simulink model "fullSys"  (R2013a)
settings: Solver=ode45  StartTime=0.0  StopTime=10.0  RelTol=1e-3
values from neighbouring files (symbols this model uses):
  g = 9.81    [init.m]
  I = diag([4.856e-3,4.856e-3,8.801e-3])    [init.m]
  m = 0.468    [init.m]
libraries: simulink x1
settings Model: Creator=vegardvo  LastModifiedBy=vegardvo

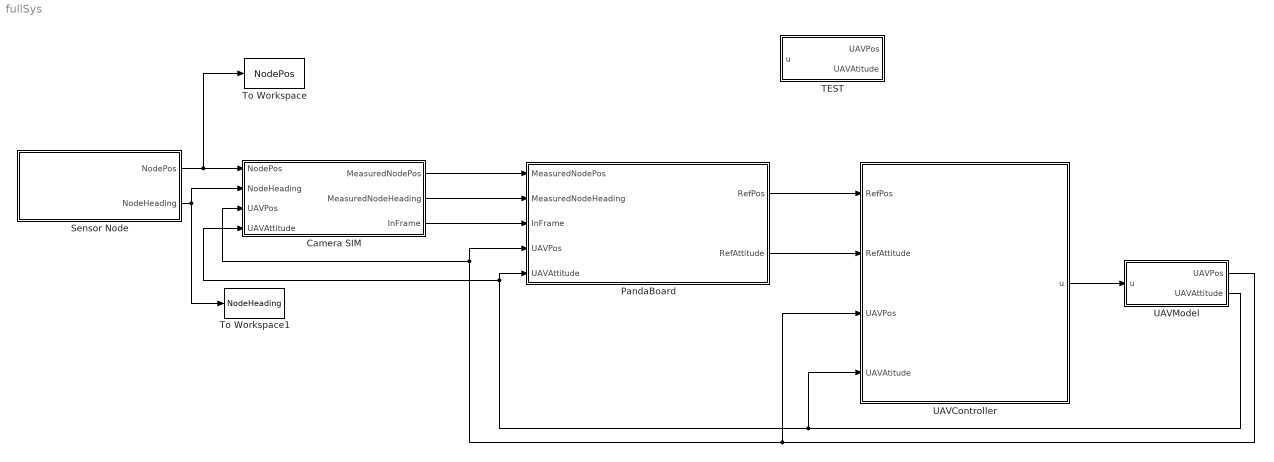
== system fullSys ==
  Camera SIM : Subsystem
  PandaBoard : Subsystem
  Sensor Node : Subsystem
  TEST : Subsystem
  To Workspace : ToWorkspace  VariableName=NodePos  SampleTime=-1  SaveFormat=Timeseries
  To Workspace1 : ToWorkspace  VariableName=NodeHeading  SampleTime=-1  SaveFormat=Timeseries
  UAVController : Subsystem
  UAVModel : Subsystem
  wires:
  Sensor Node/1(NodePos) -> Camera SIM/1(NodePos), To Workspace/1
  Camera SIM/1(MeasuredNodePos) -> PandaBoard/1(MeasuredNodePos)
  Camera SIM/3(InFrame) -> PandaBoard/3(InFrame)
  PandaBoard/1(RefPos) -> UAVController/1(RefPos)
  PandaBoard/2(RefAttitude) -> UAVController/2(RefAttitude)
  UAVController/1(u) -> UAVModel/1(u)
  UAVModel/2(UAVAttitude) -> PandaBoard/5(UAVAttitude), Camera SIM/4(UAVAttitude), UAVController/4(UAVAtitude)
  UAVModel/1(UAVPos) -> PandaBoard/4(UAVPos), Camera SIM/3(UAVPos), UAVController/3(UAVPos)
  Sensor Node/2(NodeHeading) -> To Workspace1/1, Camera SIM/2(NodeHeading)
  Camera SIM/2(MeasuredNodeHeading) -> PandaBoard/2(MeasuredNodeHeading)

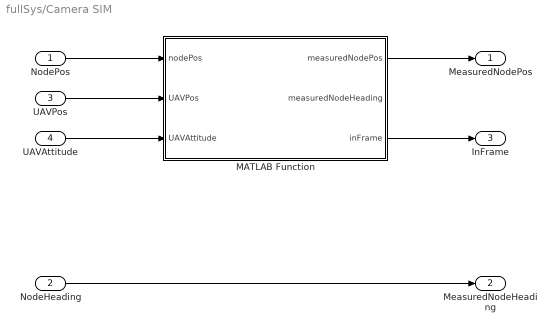
== system fullSys/Camera SIM ==
  NodePos : Inport
  NodeHeading : Inport  Port=2
  UAVPos : Inport  Port=3
  UAVAttitude : Inport  Port=4
  MATLAB Function : MATLAB Function  TreatAsAtomicUnit=on
  MeasuredNodePos : Outport
  MeasuredNodeHeading : Outport  Port=2
  InFrame : Outport  Port=3
  wires:
  NodePos/1 -> MATLAB Function/1(nodePos)
  MATLAB Function/1(measuredNodePos) -> MeasuredNodePos/1
  UAVPos/1 -> MATLAB Function/2(UAVPos)
  UAVAttitude/1 -> MATLAB Function/3(UAVAttitude)
  MATLAB Function/3(inFrame) -> InFrame/1
  NodeHeading/1 -> MeasuredNodeHeading/1

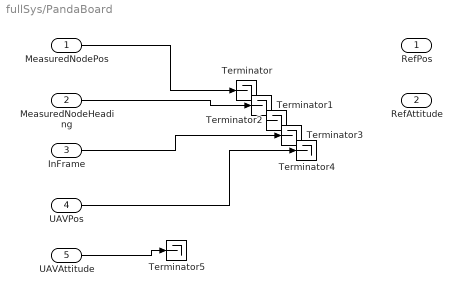
== system fullSys/PandaBoard ==
  MeasuredNodePos : Inport
  MeasuredNodeHeading : Inport  Port=2
  InFrame : Inport  Port=3
  UAVPos : Inport  Port=4
  UAVAttitude : Inport  Port=5
  Terminator{,1..5} (6 alike) : Terminator
  RefPos : Outport
  RefAttitude : Outport  Port=2
  wires:
  MeasuredNodePos/1 -> Terminator/1
  MeasuredNodeHeading/1 -> Terminator1/1
  InFrame/1 -> Terminator3/1
  UAVPos/1 -> Terminator4/1
  UAVAttitude/1 -> Terminator5/1

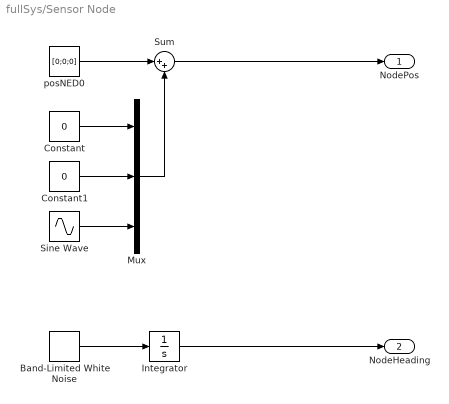
== system fullSys/Sensor Node ==
  Band-Limited White Noise : simulink/Sources/Band-Limited White Noise  Cov=[0.1]  Ts=0.1  seed=[23341]
  Constant : Constant  Value=0
  Constant1 : Constant  Value=0
  Integrator : Integrator
  Mux : Mux  Inputs=3
  Sine Wave : Sin  SampleTime=0
  Sum : Sum  Inputs=|++
  posNED0 : Constant  Value=[0;0;0]
  NodePos : Outport
  NodeHeading : Outport  Port=2
  wires:
  posNED0/1 -> Sum/1
  Sum/1 -> NodePos/1
  Mux/1 -> Sum/2
  Sine Wave/1 -> Mux/3
  Constant1/1 -> Mux/2
  Constant/1 -> Mux/1
  Band-Limited White Noise/1 -> Integrator/1
  Integrator/1 -> NodeHeading/1

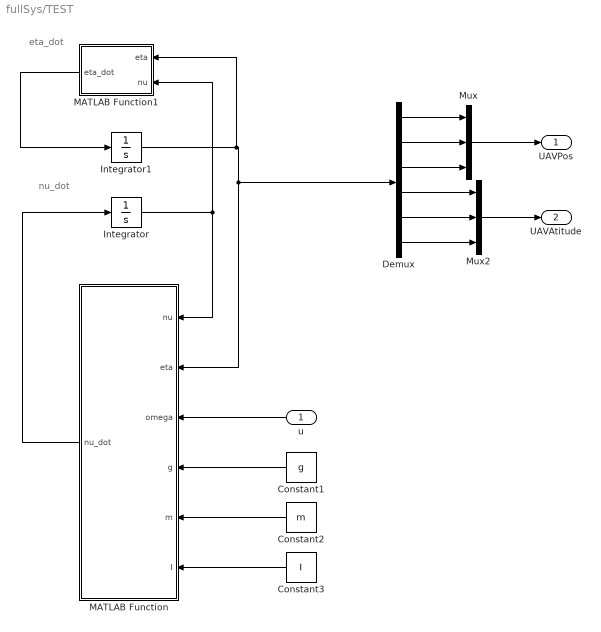
== system fullSys/TEST ==
  note: eta_dot
  note: nu_dot
  u : Inport
  Constant1 : Constant  Value=g
  Constant2 : Constant  Value=m
  Constant3 : Constant  Value=I
  Demux : Demux  Outputs=6
  Integrator : Integrator
  Integrator1 : Integrator
  MATLAB Function : MATLAB Function  TreatAsAtomicUnit=on
  MATLAB Function1 : MATLAB Function  TreatAsAtomicUnit=on
  Mux : Mux  Inputs=3
  Mux2 : Mux  Inputs=3
  UAVPos : Outport
  UAVAtitude : Outport  Port=2
  wires:
  MATLAB Function/1(nu_dot) -> Integrator/1
  Integrator/1 -> MATLAB Function/1(nu), MATLAB Function1/2(nu)
  MATLAB Function1/1(eta_dot) -> Integrator1/1
  Integrator1/1 -> MATLAB Function/2(eta), Demux/1, MATLAB Function1/1(eta)
  u/1 -> MATLAB Function/3(omega)
  Constant1/1 -> MATLAB Function/4(g)
  Constant2/1 -> MATLAB Function/5(m)
  Constant3/1 -> MATLAB Function/6(I)
  Demux/1 -> Mux/1
  Demux/2 -> Mux/2
  Demux/3 -> Mux/3
  Demux/4 -> Mux2/1
  Demux/5 -> Mux2/2
  Demux/6 -> Mux2/3
  Mux/1 -> UAVPos/1
  Mux2/1 -> UAVAtitude/1

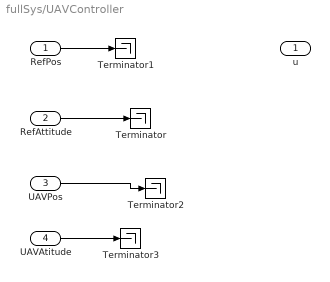
== system fullSys/UAVController ==
  RefPos : Inport
  RefAttitude : Inport  Port=2
  UAVPos : Inport  Port=3
  UAVAtitude : Inport  Port=4
  Terminator{,1..3} (4 alike) : Terminator
  u : Outport
  wires:
  RefPos/1 -> Terminator1/1
  RefAttitude/1 -> Terminator/1
  UAVPos/1 -> Terminator2/1
  UAVAtitude/1 -> Terminator3/1

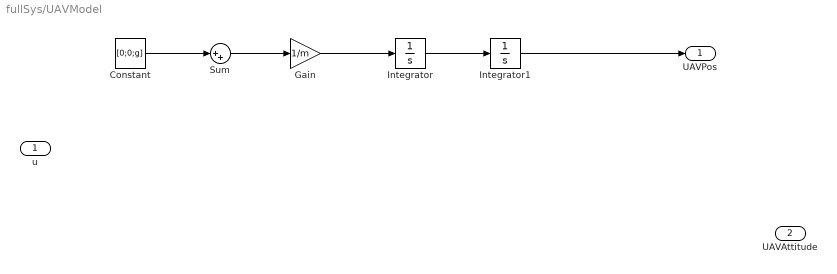
== system fullSys/UAVModel ==
  u : Inport
  Constant : Constant  Value=[0;0;g]
  Gain : Gain  Gain=1/m
  Integrator : Integrator
  Integrator1 : Integrator
  Sum : Sum  Inputs=|++
  UAVPos : Outport
  UAVAttitude : Outport  Port=2
  wires:
  Integrator1/1 -> UAVPos/1
  Integrator/1 -> Integrator1/1
  Gain/1 -> Integrator/1
  Sum/1 -> Gain/1
  Constant/1 -> Sum/1

== matlab function fullSys/Camera SIM/MATLAB Function ==
  data: nodePos input; measuredNodePos output; measuredNodeHeading output; UAVPos input; UAVAttitude input; inFrame output
function [measuredNodePos, measuredNodeHeading, inFrame] = fcn(nodePos, UAVPos, UAVAttitude)
%#codegen


% Calculate area where camera active
	% Init variables
    x_c = 320;
    y_c = 240;
    
    phi = UAVAttitude(1);
    theta = UAVAttitude(2);
    psi = UAVAttitude(3);
    height = UAVPos(3);
    
    d1 = 0;
    lengthPerPixel = 0.001328497723204;
    
    sinPhi = sin(phi);
	cosPhi = cos(phi);

	sinTheta = sin(theta);
	cosTheta = cos(theta);

	sinPsi = sin(psi);
	cosPsi = cos(psi);
    
    corners = zeros(4,2);
    x = 0;
    y = 0;
    for i = 1:4
        switch(i)
            case 1
                x = 0;
                y = 0;
            case 2
                x = 640;
                y = 0;
            case 3
                x = 640;
                y = 480;
            case 4
                x = 0;
                y = 480;
        end;
    
    deltaX = x - x_c;
 	deltaY = y - y_c;  
   
    alpha = -atan2(deltaY, -deltaX);
 	d = sqrt(deltaX^2 + deltaY^2) * lengthPerPixel;
 	beta = -atan(d);
 	sinAlpha = sin(alpha);
 	cosAlpha = cos(alpha);
 	sinBeta = sin(beta);
 	cosBeta = cos(beta);
    
    z1 = sinAlpha*sinBeta*cosPsi*cosTheta - cosAlpha*sinBeta*(-sinPsi*cosPhi + cosPsi*sinTheta*sinPhi) + cosBeta*(sinPsi*sinPhi + cosPsi*sinTheta*cosPhi);
	z2 = sinAlpha*sinBeta*sinPsi*cosTheta - cosAlpha*sinBeta*(cosPsi*cosPhi + sinPsi*sinTheta*sinPhi) + cosBeta * (-cosPsi*sinPhi + sinPsi*sinTheta*sinPhi);
 	z3 = -sinAlpha*sinBeta*sinTheta - cosAlpha*sinBeta*cosTheta*sinPhi + cosBeta*cosTheta*cosPhi;
    
    d2 = (height - d1*cosTheta*cosPhi)/z3;
    
 	corners(i,1) = d2*z1 + d1*(sinPsi*sinPhi + cosPsi*sinTheta*cosPhi);
 	corners(i,2) = d2*z2 + d1*(-cosPsi*sinPhi + sinPsi*sinTheta*cosPhi);    
    end;
 

measuredNodePos = 1; 
measuredNodeHeading = 1;
inFrame = 1;

== matlab function fullSys/TEST/MATLAB Function ==
  data: nu input; nu_dot output; eta input; omega input; g input; m input; I input
function nu_dot = fcn(nu, eta, omega, g, m, I)
%#codegen

omega_squared = omega.^2;

M_rb = [m * eye(3), zeros(3);
        zeros(3)  , I];
 
C_rb = [m*Smtrx(nu(4:6)), zeros(3);
       zeros(3), -Smtrx(I*nu(4:6))];

tau_b = [m*g*sin(eta(5));
       -m*g*cos(eta(5))*sin(eta(4));
       -m*g*cos(eta(5))*sin(eta(4));
       k*l*[-0.5, 0.5, 1, 0.5, -0.5, -1]*omega_squared;
       sqrt(3)/2 * k *l * [1,1,0,-1,-1,0]*omega_squared;
       b*[1,-1,1,-1,1,-1]*omega_squared];



nu_dot = inv(M_rb)*(tau_b - C-rb*nu));

== matlab function fullSys/TEST/MATLAB Function1 ==
  data: eta input; eta_dot output; nu input
function eta_dot = fcn(eta, nu)
%#codegen

[J, J11, J22] = eulerang(eta(4), eta(5), eta(6));

eta_dot = J*nu;
